simulink model "robot"  (R2025b)
settings: Solver=ode15s  StartTime=0.0  StopTime=10  RelTol=1e-3
settings Model: Creator=motor  LastModifiedBy=motor

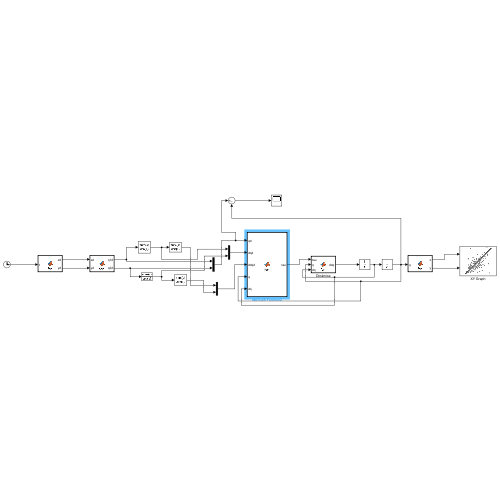
[thumbnail: Simulink's stored preview of the top-level diagram]
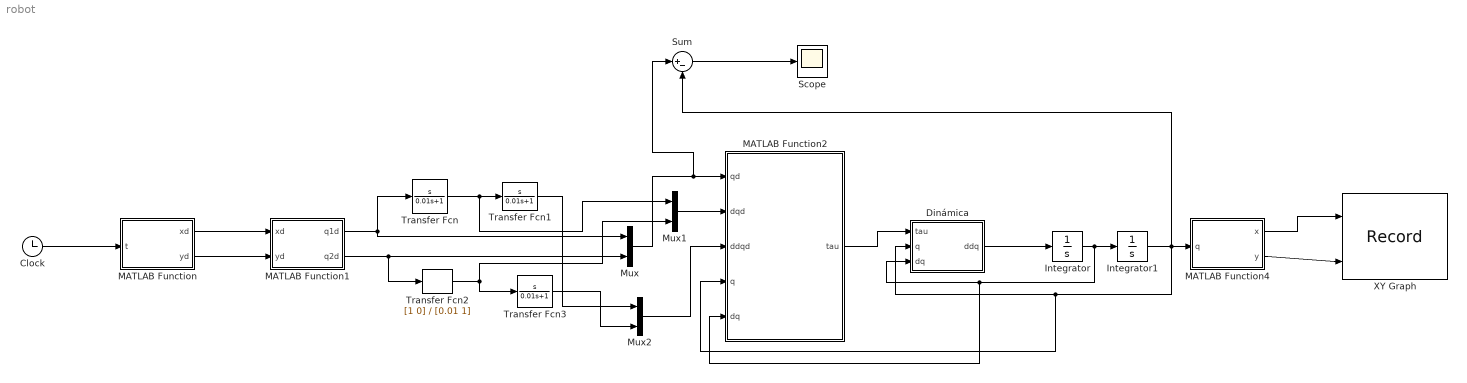
== system robot ==
  Clock : Clock
  Dinámica : MATLAB Function  TreatAsAtomicUnit=on
  Integrator : Integrator  InitialCondition=[0; 0]
  Integrator1 : Integrator  InitialCondition=[-0.25; 1.57]
  MATLAB Function : MATLAB Function  TreatAsAtomicUnit=on
  MATLAB Function1 : MATLAB Function  TreatAsAtomicUnit=on
  MATLAB Function2 : MATLAB Function  TreatAsAtomicUnit=on
  MATLAB Function4 : MATLAB Function  TreatAsAtomicUnit=on
  Mux : Mux  Inputs=2
  Mux1 : Mux  Inputs=2
  Mux2 : Mux  Inputs=2
  Scope : Scope
      settings: ActiveDisplayYMinimum=-1.85323238269956  ActiveDisplayYMaximum=0.49272579995436966
  Sum : Sum  Inputs=|+-
  Transfer Fcn{,1..3} (4 alike) : TransferFcn  Numerator=[1 0]  Denominator=[0.01 1]
  XY Graph : Record  NumPorts=2.0  FileSettingsInternal="{\"entries\":[{\"content\":{\"excelSettings\":{\"content\":{},\"type\":\"Streamout.ExcelSettings\"},\"parquetSettings\":{\"content\":{},\"type\":\"Streamout.ParquetSettings\"}},\"type\":\"Streamout.FileSettingStorage\",\"uuid\":\"\"}],\"packageUris\":[\"http:\\/\\/schema.mathworks.com\\/mf0\\/streamout_blocks\\/R2020a\"],\"version\":\"1.0\"}"  FrameSettings=[0, 0]  Layout=[1 1]  SignalsInternal="{\"entries\":[{\"content\":{\"signals\":[{\"content\":{\"blockPath\":[],\"dimensions\":[1],\"domain\":\"\",\"lineColor\":\"#a2142f\",\"plots\":[ 1 ],\"port\":1,\"sid\":[\"\"],\"signalID\":1,\"signalName\":\"MATLAB Function4:1\"},\"type\":\"RecordBlkView.Signal\",\"uuid\":\"\"},{\"content\":{\"blockPath\":[],\"dimensions\":[1],\"domain\":\"\",\"lineColor\":\"#139fff\",\"plots\":[ 1 ],\"port\":2,\"sid\":[\"\"],\"signalID\":2,\"signalName\":\"MATLAB Function4:2\"},\"type\":\"RecordBlkView.Signal\",\"uuid\":\"\"}]},\"type\":\"RecordBlkView.InputSignals\",\"uuid\":\"\"}],\"packageUris\":[\"http:\\/\\/schema.mathworks.com\\/mf0\\/streamout_blocks\\/R2020a\"],\"version\":\"1.0\"}"  VisualizationBindings="{\"xyplotplugin\":{\"info\":[{\"series\":[{\"bindingParametersList\":[{\"parameter\":\"X-Axis\",\"signalID\":1,\"signalName\":\"MATLAB Function4:1\"},{\"parameter\":\"Y-Axis\",\"signalID\":2,\"signalName\":\"MATLAB Function4:2\"}],\"seriesID\":0}],\"subplotID\":1}]}}"  CompatibilityTag=XY
  wires:
  Clock/1 -> MATLAB Function/1(t)
  MATLAB Function/1(xd) -> MATLAB Function1/1(xd)
  MATLAB Function/2(yd) -> MATLAB Function1/2(yd)
  MATLAB Function1/1(q1d) -> Mux/1, Transfer Fcn/1
  Transfer Fcn/1 -> Transfer Fcn1/1, Mux1/1
  MATLAB Function1/2(q2d) -> Transfer Fcn2/1, Mux/2
  Transfer Fcn2/1 -> Transfer Fcn3/1, Mux1/2
  Mux/1 -> Sum/1, MATLAB Function2/1(qd)
  Mux1/1 -> MATLAB Function2/2(dqd)
  Transfer Fcn3/1 -> Mux2/2
  Transfer Fcn1/1 -> Mux2/1
  Mux2/1 -> MATLAB Function2/3(ddqd)
  MATLAB Function2/1(tau) -> Dinámica/1(tau)
  Dinámica/1(ddq) -> Integrator/1
  Integrator/1 -> MATLAB Function2/5(dq), Dinámica/3(dq), Integrator1/1
  Integrator1/1 -> Sum/2, MATLAB Function4/1(q), MATLAB Function2/4(q), Dinámica/2(q)
  Sum/1 -> Scope/1
  MATLAB Function4/1(x) -> XY Graph/1
  MATLAB Function4/2(y) -> XY Graph/2

== matlab function robot/MATLAB Function1 ==
  data: xd input; q1d output; yd input; q2d output
function [q1d, q2d] = fcn(xd, yd)
    L1 = 0.4; L2 = 0.4;
    
    D = (xd^2 + yd^2 - L1^2 - L2^2) / (2*L1*L2);
    % Limitamos D entre -1 y 1 por si hay errores numéricos
    D = max(min(D, 1), -1); 
    
    q2d = acos(D); % Codo arriba
    q1d = atan2(yd, xd) - atan2(L2*sin(q2d), L1 + L2*cos(q2d));
end

== matlab function robot/MATLAB Function ==
  data: t input; xd output; yd output
function [xd, yd] = fcn(t)
    % Círculo centrado en (0.3, 0.3) con radio 0.1 en 5 segundos
    xd = 0.3 + 0.1 * cos(2*pi*t / 5);
    yd = 0.3 + 0.1 * sin(2*pi*t / 5);
end

== matlab function robot/MATLAB Function2 ==
  data: qd input; tau output; dqd input; ddqd input; q input; dq input
function tau = fcn(qd, dqd, ddqd, q, dq)
    % Parámetros
    Kp = [100 0; 0 100]; Kd = [20 0; 0 20];
    
    % Error articular
    e = qd - q;
    de = dqd - dq;
    
    % Matrices (Sustituyendo tu q2 y q1 real)
    M = [0.2933 + 0.16*cos(q(2)), 0.0533 + 0.08*cos(q(2));
         0.0533 + 0.08*cos(q(2)), 0.0533];
         
    C = [-0.08*sin(q(2))*(2*dq(1)*dq(2) + dq(2)^2);
          0.08*sin(q(2))*dq(1)^2];
          
    G = [6.867*cos(q(1)) + 1.962*cos(q(1)+q(2));
         1.962*cos(q(1)+q(2))];
         
    % Ley de control
    tau = M * (ddqd + Kp*e + Kd*de) + C + G;
end

== matlab function robot/Dinámica ==
  data: tau input; ddq output; q input; dq input
function ddq = fcn(tau, q, dq)
    % Matrices de Dinámica (tienen que declararse aquí adentro también)
    M = [0.2933 + 0.16*cos(q(2)), 0.0533 + 0.08*cos(q(2));
         0.0533 + 0.08*cos(q(2)), 0.0533];
         
    C = [-0.08*sin(q(2))*(2*dq(1)*dq(2) + dq(2)^2);
          0.08*sin(q(2))*dq(1)^2];
          
    G = [6.867*cos(q(1)) + 1.962*cos(q(1)+q(2));
         1.962*cos(q(1)+q(2))];
    
    % Despeje de la aceleración real
    ddq = M \ (tau - C - G); % Usamos "\" en vez de inv() porque a MATLAB le gusta más
end

== matlab function robot/MATLAB Function4 ==
  data: x output; q input; y output
function [x, y] = fcn(q)
    L1 = 0.4; L2 = 0.4;
    x = L1*cos(q(1)) + L2*cos(q(1)+q(2));
    y = L1*sin(q(1)) + L2*sin(q(1)+q(2));
end
